simulink model "PSO_MPPT"  (R2018a)
settings: Solver=ode23s  StartTime=0.0  StopTime=15  MaxStep=1e-4  RelTol=1e-3
undefined symbols (not defined in the file): sigbuilder_block
libraries: powerlib x12, re_lib x3, powerlib_meascontrol x1
settings Model: Creator=Mahesh Krishna  LastModifiedBy=AJAY
settings OptimizationCC: EfficientMapNaN2IntZero=off  LifeSpan=inf
settings DebuggingCC: SFExecutionAtInitializationDiag=none
settings HardwareCC: TargetBitPerPointer=64  TargetBitPerSizeT=64  TargetBitPerPtrDiffT=64  TargetLongLongMode=on  TargetIntDivRoundTo=Zero  TargetEndianess=LittleEndian  TargetWordSize=64  TargetHWDeviceType=MATLAB Host  ProdEqTarget=off
settings CodeAppCC: MaxIdLength=128  StateflowObjectComments=on
settings GRTTargetCC: TargetLangStandard=C89/C90 (ANSI)  CombineOutputUpdateFcns=off  GRTInterface=on
settings SimscapeCC: SimscapeNormalizeSystem=off

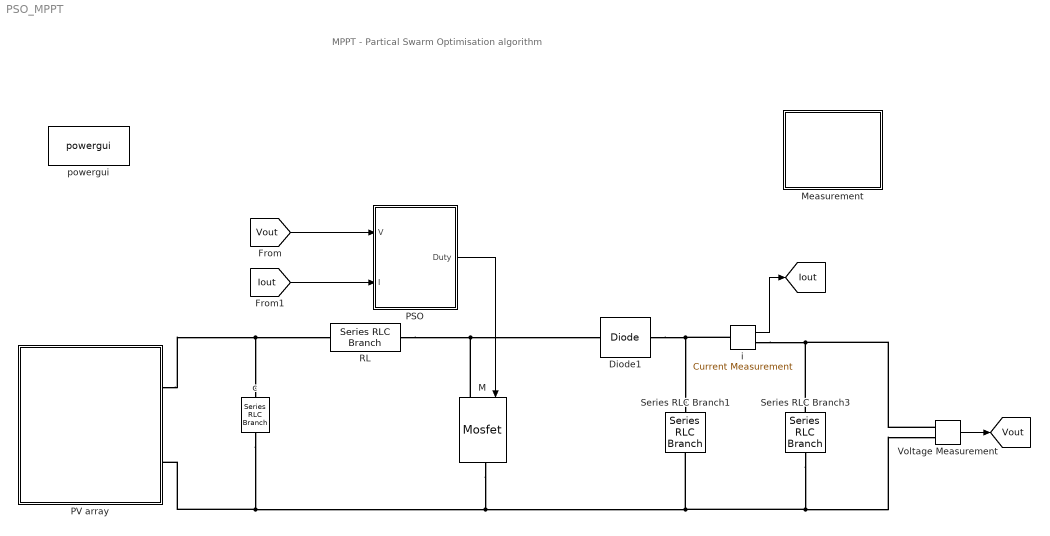
== system PSO_MPPT ==
  note: MPPT - Partical Swarm Optimisation algorithm
  Diode1 : powerlib/Power Electronics/Diode  Ron=1e-3  Lon=0  Vf=0  IC=0  UseSnubber=off  Rs=inf  Cs=inf  Measurements=off
  M : powerlib/Power Electronics/Mosfet  Ron=1e-3  Lon=0  Rd=1e-3  Vfd=0  IC=0  Rs=inf  Cs=inf  Measurements=off
  Measurement : Subsystem
  PSO : Subsystem
  PV array : Subsystem
  RL : powerlib/Elements/Series RLC Branch  LConnTagsString=__new0  RConnTagsString=__new0  BranchType=L  Resistance=1e-3  Inductance=300e-6  SetiL0=off  InitialCurrent=0  Capacitance=1e-6  Setx0=off  InitialVoltage=0  Measurements=None
  Series RLC Branch1 : powerlib/Elements/Series RLC Branch  LConnTagsString=__new0  RConnTagsString=__new0  BranchType=C  Resistance=1e-4  Inductance=200e-6  SetiL0=off  InitialCurrent=0  Capacitance=1000e-6  Setx0=off  InitialVoltage=40  Measurements=None
  Series RLC Branch3 : powerlib/Elements/Series RLC Branch  LConnTagsString=__new0  RConnTagsString=__new0  BranchType=R  Resistance=50  Inductance=200e-6  SetiL0=off  InitialCurrent=0  Capacitance=1000e-6  Setx0=off  InitialVoltage=40  Measurements=None
  Voltage Measurement : powerlib/Measurements/Voltage Measurement  PhasorSimulation=off  OutputType=Magnitude  PSBequivalent=0
  c : powerlib/Elements/Series RLC Branch  LConnTagsString=__new0  RConnTagsString=__new0  BranchType=C  Resistance=1e-3  Inductance=250e-6  SetiL0=off  InitialCurrent=0  Capacitance=100e-6  Setx0=off  InitialVoltage=0  Measurements=None
  i : powerlib/Measurements/Current Measurement  PhasorSimulation=off  OutputType=Magnitude  PSBequivalent=0
  powergui : powerlib/powergui  Priority=1  SimulationMode=Continuous  SampleTime=50e-6  frequency=60  Iterations=50  frequencyindice=0  Pbase=100e6  ErrMax=1e-4  UnitsV=kV  UnitsW=MW  buscounter=0  FunctionMessages=off  echomessages=off  EnableUseOfTLC=off  CurrentSourceSwitches=off  DisableSnubberDevices=off  DisableRonSwitches=off  DisableVfSwitches=off  DisplayEquations=off  SolverType=Tustin/Backward Euler (TBE)  Interpol=off  ExternalGateDelay=off  methode=off  Ts=100  x0status=blocks  SPID=on  SwTol=0  HookPort=off  RestoreLinks=warning  ResistiveCurrentMeasurement=off  Frange=[0:2:500]  Ylog=off  Xlog=on  ShowGrid=off  save=off  variable=ZData  structure=0  ZoomFFT=off  StartTime=0.0  cycles=1  DisplayStyle=1  fundamental=60  FreqAxis=off  MaxFrequency=1000  frequencyindicesteady=1  RmsSteady=1  display=off
  tag scope: Iout=global, Vout=global
  wires:
  Voltage Measurement/1 -> [Vout]
  i/1 -> [Iout]
  [Vout] -> PSO/1(V)
  [Iout] -> PSO/2("I ")
  PSO/1(Duty) -> M/1
  connections:
  i/RConn1 -- Series RLC Branch3/LConn1 -- Voltage Measurement/LConn1
  Series RLC Branch1/RConn1 -- c/RConn1 -- PV array/RConn2 -- M/RConn1 -- Series RLC Branch3/RConn1 -- Voltage Measurement/LConn2
  Diode1/RConn1 -- Series RLC Branch1/LConn1 -- i/LConn1
  M/LConn1 -- Diode1/LConn1 -- RL/RConn1
  PV array/RConn1 -- RL/LConn1 -- c/LConn1

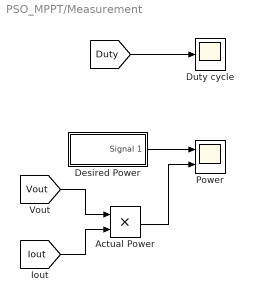
== system PSO_MPPT/Measurement ==
  Actual Power : Product
  Desired Power : Subsystem  Tag=STV Subsys  LoadFcn=sigbuilder_block('load');  StartFcn=sigbuilder_block('start');  StopFcn=sigbuilder_block('stop');  ClipboardFcn=sigbuilder_block('clipboard');  mask(Sigbuilder block){tuvar=[0:10]}
      mask help: Simulink:masks:SigbuilderBlock_MD
      mask init:
      | if ~strcmp(get_param(bdroot(gcbh),'SimulationStatus'),'stopped') tuvar = sigbuilder_block('maskInit'); end
      settings: CopyFcn=sigbuilder_block('copy');  DeleteFcn=sigbuilder_block('delete');  ModelCloseFcn=sigbuilder_block('modelClose');  PreSaveFcn=sigbuilder_block('preSave');  PauseFcn=sigbuilder_block('pause');  ContinueFcn=sigbuilder_block('continue');  NameChangeFcn=sigbuilder_block('namechange');  OpenFcn=sigbuilder_block('open',[437.25 153 550.5 359.25 ]);  CloseFcn=sigbuilder_block('close');
      mask Display: plot(0, 0, 100, 100,[2, 2, 32, 32, 2], [68, 8, 8, 68, 68],[32, 2], [38, 38], [32, 19, 2],[53, 60, 44], [32, 17, 17, 2],[16, 16, 31, 31]);txt = getActiveGroup(gcbh);text(2, 100, txt,'verticalAlignment', 'top');
  Duty cycle : Scope
  Power : Scope  NumInputPorts=2
  wires:
  [Iout] -> Actual Power/2
  [Vout] -> Actual Power/1
  Actual Power/1 -> Power/2
  [Duty] -> Duty cycle/1
  Desired Power/1(Signal 1) -> Power/1

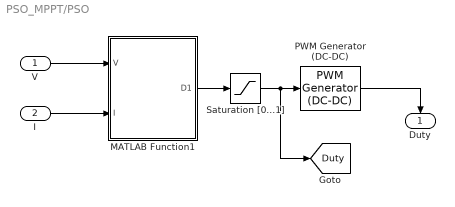
== system PSO_MPPT/PSO ==
  V : Inport
  "I " : Inport  Port=2
  MATLAB Function1 : MATLAB Function  TreatAsAtomicUnit=on
  PWM Generator (DC-DC) : powerlib_meascontrol/Pulse & Signal Generators/PWM Generator (DC-DC)  Fsw=50e3  Ts=0
  Saturation [0...1] : Saturate  UpperLimit=1  LowerLimit=0
  Duty : Outport
  tag scope: Duty=global
  wires:
  Saturation [0...1]/1 -> [Duty], PWM Generator (DC-DC)/1
  "I "/1 -> MATLAB Function1/2(I)
  MATLAB Function1/1(D1) -> Saturation [0...1]/1
  V/1 -> MATLAB Function1/1(V)
  PWM Generator (DC-DC)/1 -> Duty/1

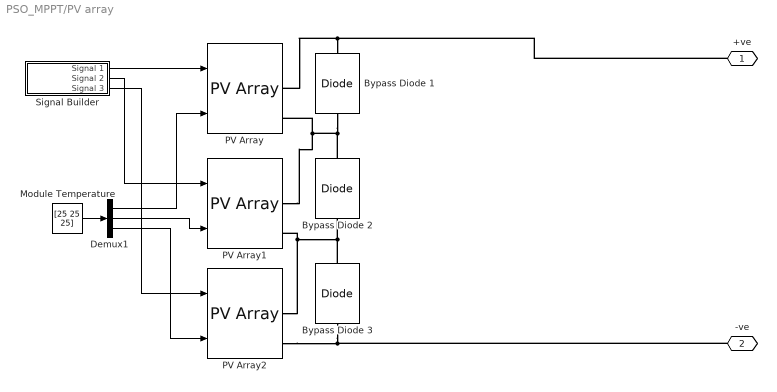
== system PSO_MPPT/PV array ==
  Bypass Diode 1 : powerlib/Power Electronics/Diode  Ron=0.001  Lon=0  Vf=0.8  IC=0  UseSnubber=off  Rs=500  Cs=250e-9  Measurements=off
  Bypass Diode 2 : powerlib/Power Electronics/Diode  Ron=0.001  Lon=0  Vf=0.8  IC=0  UseSnubber=off  Rs=500  Cs=250e-9  Measurements=off
  Bypass Diode 3 : powerlib/Power Electronics/Diode  Ron=0.001  Lon=0  Vf=0.8  IC=0  UseSnubber=off  Rs=500  Cs=250e-9  Measurements=off
  Demux1 : Demux  Outputs=3
  Module Temperature : Constant  Value=[25 25 25]
  PV Array : re_lib/Solar/PV Array  Npar=1  Nser=1  PlotType=array @ 1000 W/m2 & specified temperatures  S_vec="[ 1000  500  100 ]"  Temp_C_vec="[ 45 25  ]"  ModuleName=User-defined  PlotWhenSelected=off  Pm=39.96  Ncell=60  Voc=21.8  Isc=2.41  Vm=18  Im=2.22  beta_Voc_pc=-0.36099  alpha_Isc_pc=0.102  beta_Voc=-0.078696  alpha_Isc=0.0024582  IL=2.4478  I0=8.8348e-11  nI=0.58954  Rsh=161.0785  Rs=0.47771  BAL=on  Tc=1e-6  Tfilter=5e-5
  PV Array1 : re_lib/Solar/PV Array  Npar=1  Nser=1  PlotType=array @ 1000 W/m2 & specified temperatures  S_vec="[ 1000  500  100 ]"  Temp_C_vec="[ 45 25  ]"  ModuleName=User-defined  PlotWhenSelected=off  Pm=39.96  Ncell=60  Voc=21.8  Isc=2.41  Vm=18  Im=2.22  beta_Voc_pc=-0.36099  alpha_Isc_pc=0.102  beta_Voc=-0.078696  alpha_Isc=0.0024582  IL=2.4478  I0=8.8348e-11  nI=0.58954  Rsh=161.0785  Rs=0.47771  BAL=on  Tc=1e-6  Tfilter=5e-5
  PV Array2 : re_lib/Solar/PV Array  Npar=1  Nser=1  PlotType=array @ 1000 W/m2 & specified temperatures  S_vec="[ 1000  500  100 ]"  Temp_C_vec="[ 45 25  ]"  ModuleName=User-defined  PlotWhenSelected=off  Pm=39.96  Ncell=60  Voc=21.8  Isc=2.41  Vm=18  Im=2.22  beta_Voc_pc=-0.36099  alpha_Isc_pc=0.102  beta_Voc=-0.078696  alpha_Isc=0.0024582  IL=2.4478  I0=8.8348e-11  nI=0.58954  Rsh=161.0785  Rs=0.47771  BAL=on  Tc=1e-6  Tfilter=5e-5
  Signal Builder : Subsystem  Tag=STV Subsys  LoadFcn=sigbuilder_block('load');  StartFcn=sigbuilder_block('start');  StopFcn=sigbuilder_block('stop');  ClipboardFcn=sigbuilder_block('clipboard');  mask(Sigbuilder block){tuvar=[0:10]}
      mask help: Simulink:masks:SigbuilderBlock_MD
      mask init:
      | if ~strcmp(get_param(bdroot(gcbh),'SimulationStatus'),'stopped') tuvar = sigbuilder_block('maskInit'); end
      settings: CopyFcn=sigbuilder_block('copy');  DeleteFcn=sigbuilder_block('delete');  ModelCloseFcn=sigbuilder_block('modelClose');  PreSaveFcn=sigbuilder_block('preSave');  PauseFcn=sigbuilder_block('pause');  ContinueFcn=sigbuilder_block('continue');  NameChangeFcn=sigbuilder_block('namechange');  OpenFcn=sigbuilder_block('open',[437.25 153 550.5 359.25 ]);  CloseFcn=sigbuilder_block('close');
      mask Display: plot(0, 0, 100, 100,[2, 2, 32, 32, 2], [68, 8, 8, 68, 68],[32, 2], [38, 38], [32, 19, 2],[53, 60, 44], [32, 17, 17, 2],[16, 16, 31, 31]);txt = getActiveGroup(gcbh);text(2, 100, txt,'verticalAlignment', 'top');
  " +ve" : PMIOPort  Side=Right
  -ve : PMIOPort  Port=2  Side=Right
  wires:
  Signal Builder/2(Signal 2) -> PV Array1/1
  Module Temperature/1 -> Demux1/1
  Signal Builder/3(Signal 3) -> PV Array2/1
  Demux1/2 -> PV Array1/2
  Signal Builder/1(Signal 1) -> PV Array/1
  Demux1/1 -> PV Array/2
  Demux1/3 -> PV Array2/2
  connections:
  PV Array1/RConn2 -- Bypass Diode 3/RConn1 -- Bypass Diode 2/LConn1 -- PV Array2/RConn1
  PV Array2/RConn2 -- -ve/RConn1 -- Bypass Diode 3/LConn1
  PV Array/RConn2 -- Bypass Diode 2/RConn1 -- Bypass Diode 1/LConn1 -- PV Array1/RConn1
  PV Array/RConn1 -- " +ve"/RConn1 -- Bypass Diode 1/RConn1

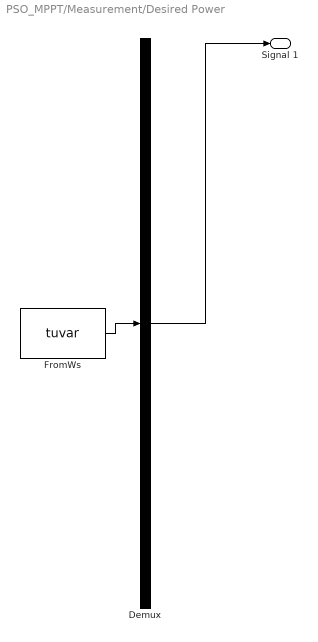
== system PSO_MPPT/Measurement/Desired Power ==
  Demux : Demux  Tag=STV Demux  Outputs=1
  FromWs : FromWorkspace  Tag=STV FromWs  VariableName=tuvar  SampleTime=0
      SigBuilderData=|
      | common.afterFinalStr = 'Extrapolate'
      | common.sampleTime = 0
      | dataSet.timeRange = [0 15]
      | dataSet.name = 'Group 1'
      | sbobj.Groups.Name = 'Group 1'
      | sbobj.Groups.Signals.Name = 'Signal 1'
      | sbobj.Groups.Signals.XData = [0 4 4 8 8 15]
      | sbobj.Groups.Signals.YData = [78.5 78.5 65.5 65.5 36.2 36.2]
      | sbobj.Groups.TimeRange = [0 15]
  Signal 1 : Outport  Tag=STV Outport
  wires:
  Demux/1 -> Signal 1/1
  FromWs/1 -> Demux/1

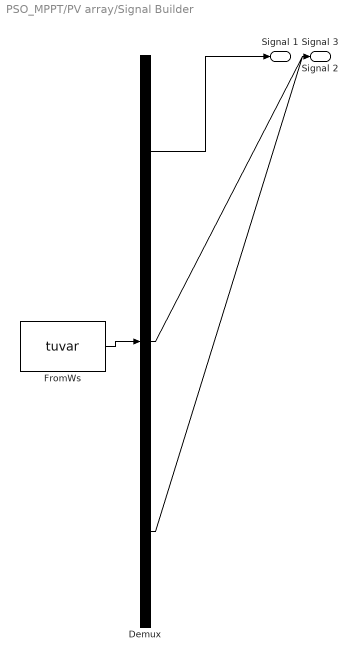
== system PSO_MPPT/PV array/Signal Builder ==
  Demux : Demux  Tag=STV Demux  Outputs=3
  FromWs : FromWorkspace  Tag=STV FromWs  VariableName=tuvar  SampleTime=0
      SigBuilderData=|
      | common.afterFinalStr = 'Extrapolate'
      | common.sampleTime = 0
      | dataSet.timeRange = [0 15]
      | dataSet.name = 'Group 1'
      | sbobj.Groups.Name = 'Group 1'
      | sbobj.Groups.Signals(1).Name = 'Signal 1'
      | sbobj.Groups.Signals(1).XData = [0 4 4 8 8 15]
      | sbobj.Groups.Signals(1).YData = [1000 1000 800 800 1000 1000]
      | sbobj.Groups.Signals(2).Name = 'Signal 2'
      | sbobj.Groups.Signals(2).XData = [0 4 4 8 8 15]
      | sbobj.Groups.Signals(2).YData = [800 800 1000 1000 300 300]
      | sbobj.Groups.Signals(3).Name = 'Signal 3'
      | sbobj.Groups.Signals(3).XData = [0 4 4 8 8 15]
      | sbobj.Groups.Signals(3).YData = [600 600 300 300 100 100]
      | sbobj.Groups.TimeRange = [0 15]
  Signal 1 : Outport  Tag=STV Outport
  Signal 2 : Outport  Tag=STV Outport  Port=2
  Signal 3 : Outport  Tag=STV Outport  Port=3
  wires:
  Demux/1 -> Signal 1/1
  FromWs/1 -> Demux/1
  Demux/2 -> Signal 2/1
  Demux/3 -> Signal 3/1

== matlab function PSO_MPPT/PSO/MATLAB Function1 ==
  settings: updateMethod=DISCRETE  sampleTime=1e-4
  data: V input; D1 output; I input
function D1 = PSO(V,I)
persistent q w P initialization itteration power dcurrent counter current_dutycycl velocity current_power local_best_power local_best_dutycycl globl_best_dutycycl global_best_power

D1=0.05;

if isempty(q)
    q=1;
end

if isempty(w)
    w=1;
end

if isempty(P)
    P=zeros(1,3);
end

if isempty(initialization)
    initialization=1;
end

if isempty(itteration)
    itteration=0;
end

if isempty(power)
    power=0;
end

if isempty(current_dutycycl)
    current_dutycycl=zeros(1,3);
end
if isempty(velocity)
    velocity=zeros(1,3);
end
if isempty(current_power)
    current_power=zeros(1,3);
end
if isempty(local_best_power)
    local_best_power=zeros(1,3);
end
if isempty(local_best_dutycycl)
    local_best_dutycycl=zeros(1,3);
end
if isempty(globl_best_dutycycl)
    globl_best_dutycycl=0;
end

if isempty(global_best_power)
    global_best_power=0;
end

if(isempty(dcurrent))
    dcurrent=0;
end

if isempty(counter)
    counter = 0;
end

if(counter>=1 && counter<800)
    D1=dcurrent;
    counter=counter+1;
    return;
end
counter = 0;

e= 0.4;
c1= 0.8;
c2=1.2;
R1=0.25;
R2=0.25;
    
%INITIALIZATION
if itteration<13
    if q==1
    %random dutycycle-1
        if w==1
            if initialization == 1
                current_dutycycl(q)=0.05; %generate random duty value
                velocity(:,q)= 0;
            else
                velocity(:,q)=e *velocity(:,q)+ c1*(R1.*(local_best_dutycycl(:,q)-current_dutycycl(:,q))) +c2*(R2.*(globl_best_dutycycl-current_dutycycl(:,q)));
            end
            current_dutycycl(q)=current_dutycycl(q)+velocity(:,q);
            D1 = current_dutycycl(q);
            dcurrent=current_dutycycl(q);
            counter=1;
            w=2;
            return;
        end
        D1=dcurrent;
        P(:,1)=V*I;
        if P(:,q)> local_best_power(:,q)
            local_best_dutycycl(:,q)= current_dutycycl(:,q);
            local_best_power(:,q)=P(:,q);
        end
        if local_best_power(:,q)> global_best_power
            global_best_power = local_best_power(:,q);
            globl_best_dutycycl=local_best_dutycycl(:,q);
        end
        q=q+1;
    elseif q==2
        %random dutycycle-2
        if w==2      
            if initialization == 1
                current_dutycycl(q)=0.40; %generate random duty value
                velocity(:,q)= 0;
            else
                velocity(:,q)=e *velocity(:,q)+ c1*(R1.*(local_best_dutycycl(:,q)-current_dutycycl(:,q))) +c2*(R2.*(globl_best_dutycycl-current_dutycycl(:,q)));
            end
            current_dutycycl(q)=current_dutycycl(q)+velocity(:,q);
            D1 = current_dutycycl(q);
            dcurrent=current_dutycycl(q);
            counter=1;
            w=3;
            return;
        end
        D1=dcurrent;
        P(:,2)=V*I;
        if P(:,q)> local_best_power(:,q)
            local_best_dutycycl(:,q)= current_dutycycl(:,q);
            local_best_power(:,q)=P(:,q);
        end
        if local_best_power(:,q)> global_best_power
            global_best_power = local_best_power(:,q);
            globl_best_dutycycl=local_best_dutycycl(:,q);
        end
        q=q+1;
    else
        %random dutycycle-3
        if w==3
            if initialization == 1
                current_dutycycl(q)=0.95; %generate random duty value
                velocity(:,q)= 0;
            else
                velocity(:,q)=e *velocity(:,q)+ c1*(R1.*(local_best_dutycycl(:,q)-current_dutycycl(:,q))) +c2*(R2.*(globl_best_dutycycl-current_dutycycl(:,q)));
            end
            current_dutycycl(q)=current_dutycycl(q)+velocity(:,q);
            D1 = current_dutycycl(q);
            dcurrent=current_dutycycl(q);
            counter=1;
            w=1;
            return;
        end
        D1=dcurrent;
        P(:,3)=V*I;
        if P(:,q)> local_best_power(:,q)
            local_best_dutycycl(:,q)= current_dutycycl(:,q);
            local_best_power(:,q)=P(:,q);
        end
        if local_best_power(:,q)> global_best_power
            global_best_power = local_best_power(:,q);
            globl_best_dutycycl=local_best_dutycycl(:,q);
        end
        q=1;
        initialization =2;
        itteration = itteration +1;
    end
else
    power = V*I;
    if (global_best_power - power)>5
        q=1;
        w=1;
        initialization = 1;
        itteration = 1;
        dcurrent = 0.05;
        counter = 1;
        local_best_power=zeros(1,3);
        local_best_dutycycl=zeros(1,3);
        globl_best_dutycycl=0;
        global_best_power=0;
        power = 0;
    else
        D1 = globl_best_dutycycl;
    end        
end
